simulink model "Fan_on_off"  (R2016b)
settings: Solver=FixedStepDiscrete  StartTime=0.0  StopTime=10.0  FixedStep=0.1  RelTol=1e-3  EnableMultiTasking=on
settings Model: Creator=Saher Ghanem  LastModifiedBy=Saher Ghanem
settings SolverCC: AutoInsertRateTranBlk=on
settings DataIOCC: LimitDataPoints=on
settings OptimizationCC: LifeSpan=inf
settings DebuggingCC: AllowSymbolicDim=off  SFUnexpectedBacktrackingDiag=warning  SFNoUnconditionalDefaultTransitionDiag=warning  SFExecutionAtInitializationDiag=none
settings GRTTargetCC: TargetLangStandard=C89/C90 (ANSI)  GeneratePreprocessorConditionals=Disable all
settings ConfigComp: CovMetricSettings=dw  CovHtmlReporting=on  CovSaveCumulativeToWorkspaceVar=on  CovSaveSingleToWorkspaceVar=on  CovExternalEMLEnable=off  CovSFcnEnable=off

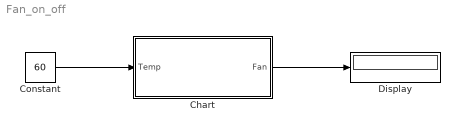
== system Fan_on_off ==
  Chart : Stateflow chart  TreatAsAtomicUnit=on
  Constant : Constant  Value=60
  Display : Display
  wires:
  Constant/1 -> Chart/1(Temp)
  Chart/1(Fan) -> Display/1

== stateflow chart Fan_on_off/Chart ==
  state Fan_State2
    Fan=1;
  state Fan_State1
    Fan=0;
  Fan_State1 -> Fan_State2 : [Temp>=50]
  (default) -> Fan_State1
  Fan_State2 -> Fan_State1 : [Temp<50]
  data: Temp input double; Fan output double
